simulink model "Project7_Trial"  (R2021b)
settings: Solver=VariableStepAuto  StartTime=0.0  StopTime=Sim_Time  RelTol=1e-3
values from neighbouring files (symbols this model uses):
  b = 10    [Project7_Run.m]
  k = 20    [Project7_Run.m]
  Kd = 50    [Project7_Run.m]
  Ki = 300    [Project7_Run.m]
  Kp = 350    [Project7_Run.m]
  M = 1    [Project7_Run.m]
settings Model: Creator=rohitkharat  LastModifiedBy=rohitkharat

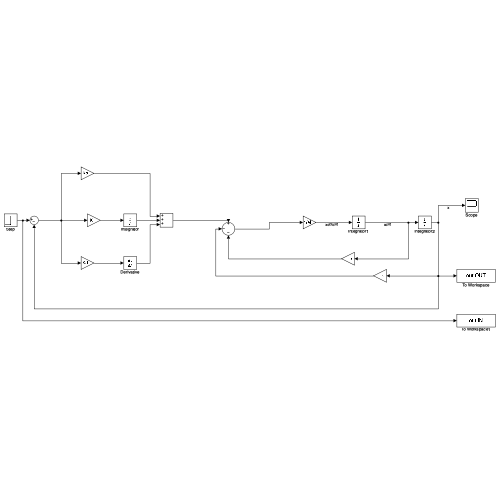
[thumbnail: Simulink's stored preview of the top-level diagram]
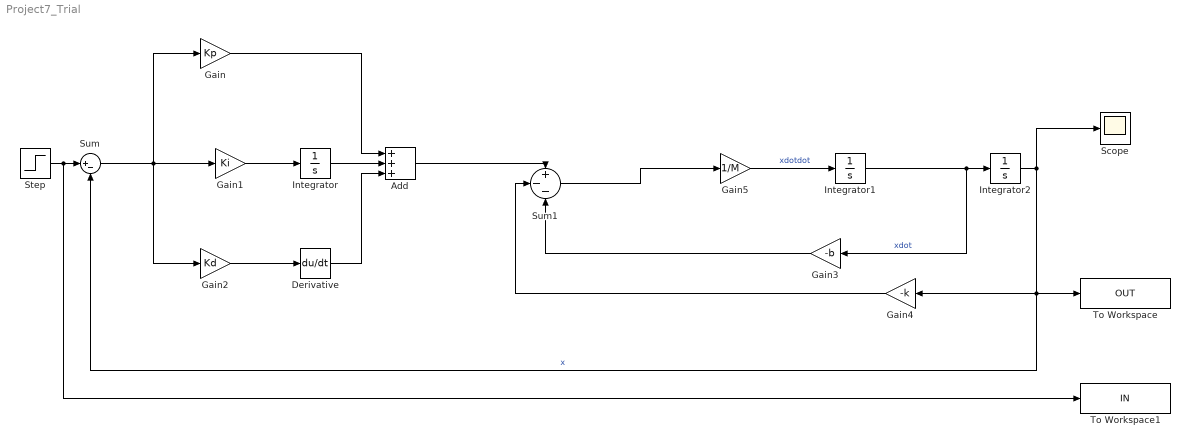
== system Project7_Trial ==
  Add : Sum  Inputs=+++
  Derivative : Derivative
  Gain : Gain  Gain=Kp
  Gain1 : Gain  Gain=Ki
  Gain2 : Gain  Gain=Kd
  Gain3 : Gain  Gain=-b
  Gain4 : Gain  Gain=-k
  Gain5 : Gain  Gain=1/M
  Integrator : Integrator
  Integrator1 : Integrator
  Integrator2 : Integrator
  Scope : Scope
  Step : Step  SampleTime=0
  Sum : Sum  Inputs=|+-
  Sum1 : Sum  Inputs=+--
  To Workspace : ToWorkspace  VariableName=OUT  SaveFormat=Timeseries  SampleTime=-1
  To Workspace1 : ToWorkspace  VariableName=IN  SaveFormat=Timeseries  SampleTime=-1
  wires:
  Sum/1 -> Gain2/1, Gain1/1, Gain/1
  Gain/1 -> Add/1
  Derivative/1 -> Add/3
  Gain1/1 -> Integrator/1
  Integrator/1 -> Add/2
  Gain2/1 -> Derivative/1
  Step/1 -> To Workspace1/1, Sum/1
  Gain4/1 -> Sum1/2
  Gain3/1 -> Sum1/3
  Integrator2/1 -> To Workspace/1, Gain4/1, Sum/2, Scope/1  "x"
  Integrator1/1 -> Gain3/1, Integrator2/1  "xdot"
  Gain5/1 -> Integrator1/1  "xdotdot"
  Sum1/1 -> Gain5/1
  Add/1 -> Sum1/1
